simulink model "tapped_delay_line2"  (R2019a)
settings: Solver=FixedStepAuto  StartTime=0.0  StopTime=endtime  FixedStep=0.001  RelTol=1e-3
undefined symbols (not defined in the file or in its folder): Gpd, K
settings Model: Creator=chris  LastModifiedBy=chris

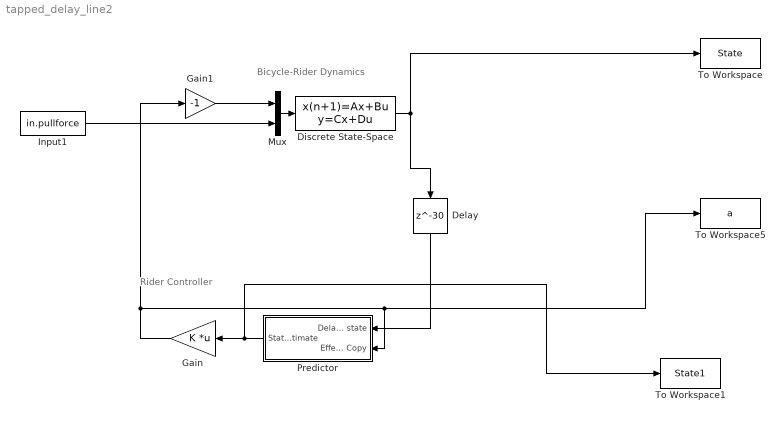
== system tapped_delay_line2 ==
  note: Rider Controller
  note: Bicycle-Rider Dynamics
  Delay : Delay  DelayLength=30  InitialCondition=0
  Discrete State-Space : DiscreteStateSpace  A=Gpd.A  B=Gpd.B  C=Gpd.C  D=Gpd.D  SampleTime=-1
  Gain : Gain  Gain=K  Multiplication=Matrix(K*u) (u vector)
  Gain1 : Gain  Gain=-1
  Input1 : FromWorkspace  VariableName=in.pullforce  SampleTime=0
  Mux : Mux  Inputs=2
  "Predictor " : Subsystem
  To Workspace : ToWorkspace  VariableName=State  SampleTime=-1
  To Workspace1 : ToWorkspace  VariableName=State1  SampleTime=-1
  To Workspace5 : ToWorkspace  VariableName=a  SampleTime=-1
  wires:
  Discrete State-Space/1 -> Delay/1, To Workspace/1
  Mux/1 -> Discrete State-Space/1
  Gain1/1 -> Mux/1
  Input1/1 -> Mux/2
  Gain/1 -> To Workspace5/1, "Predictor "/2("Efference Copy "), Gain1/1
  "Predictor "/1("State Estimate ") -> To Workspace1/1, Gain/1
  Delay/1 -> "Predictor "/1("Delayed state ")

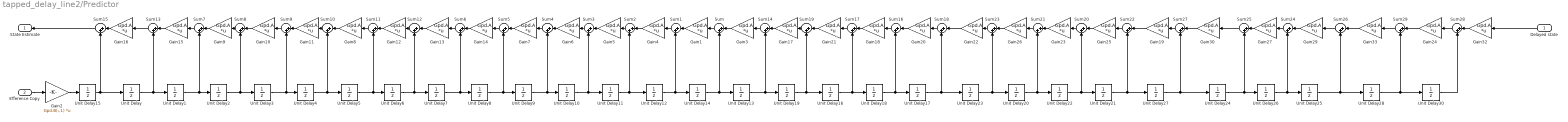
== system tapped_delay_line2/Predictor  ==
  "Delayed state " : Inport
  "Efference Copy " : Inport  Port=2
  Gain{1,3..27,29..30,32..33} (30 alike) : Gain  Gain=Gpd.A  Multiplication=Matrix(K*u) (u vector)
  Gain2 : Gain  Gain=Gpd.B(:,1)  Multiplication=Matrix(K*u) (u vector)
  Sum{,1..29} (30 alike) : Sum  Inputs=|++
  Unit Delay{,1..28,30} (30 alike) : UnitDelay  SampleTime=-1  HasFrameUpgradeWarning=on
  "State Estimate " : Outport
  wires:
  "Efference Copy "/1 -> Gain2/1
  Unit Delay/1 -> Sum13/2, Unit Delay1/1
  Unit Delay1/1 -> Sum7/2, Unit Delay2/1
  Unit Delay2/1 -> Sum8/2, Unit Delay3/1
  Unit Delay3/1 -> Sum9/2, Unit Delay4/1
  Unit Delay4/1 -> Sum10/2, Unit Delay5/1
  Unit Delay5/1 -> Sum11/2, Unit Delay6/1
  Unit Delay6/1 -> Sum12/2, Unit Delay7/1
  Unit Delay7/1 -> Sum6/2, Unit Delay8/1
  Unit Delay8/1 -> Unit Delay9/1, Sum5/2
  Unit Delay9/1 -> Sum4/2, Unit Delay10/1
  Unit Delay10/1 -> Sum3/2, Unit Delay11/1
  Unit Delay11/1 -> Unit Delay12/1, Sum2/2
  Unit Delay14/1 -> Unit Delay13/1, Sum/2
  Unit Delay12/1 -> Sum1/2, Unit Delay14/1
  Gain1/1 -> Sum1/1
  Sum/1 -> Gain1/1
  Gain3/1 -> Sum/1
  Sum1/1 -> Gain4/1
  Sum2/1 -> Gain5/1
  Gain4/1 -> Sum2/1
  Sum3/1 -> Gain6/1
  Gain5/1 -> Sum3/1
  Sum4/1 -> Gain7/1
  Gain6/1 -> Sum4/1
  Sum5/1 -> Gain14/1
  Gain7/1 -> Sum5/1
  Sum6/1 -> Gain13/1
  Gain14/1 -> Sum6/1
  Sum7/1 -> Gain15/1
  Gain9/1 -> Sum7/1
  Sum8/1 -> Gain9/1
  Gain10/1 -> Sum8/1
  Sum9/1 -> Gain10/1
  Gain11/1 -> Sum9/1
  Sum10/1 -> Gain11/1
  Gain8/1 -> Sum10/1
  Sum11/1 -> Gain8/1
  Gain12/1 -> Sum11/1
  Sum12/1 -> Gain12/1
  Gain13/1 -> Sum12/1
  Sum13/1 -> Gain16/1
  Gain15/1 -> Sum13/1
  Unit Delay13/1 -> Sum14/2, Unit Delay19/1
  Sum14/1 -> Gain3/1
  Gain17/1 -> Sum14/1
  Unit Delay15/1 -> Unit Delay/1, Sum15/2
  Gain2/1 -> Unit Delay15/1
  Gain16/1 -> Sum15/1
  Sum15/1 -> "State Estimate "/1
  Unit Delay18/1 -> Unit Delay17/1, Sum16/2
  Gain22/1 -> Sum18/1
  Unit Delay16/1 -> Sum17/2, Unit Delay18/1
  Gain18/1 -> Sum17/1
  Sum17/1 -> Gain21/1
  Sum16/1 -> Gain18/1
  Gain20/1 -> Sum16/1
  Sum18/1 -> Gain20/1
  Unit Delay19/1 -> Unit Delay16/1, Sum19/2
  Sum19/1 -> Gain17/1
  Gain21/1 -> Sum19/1
  Sum20/1 -> Gain23/1
  Sum21/1 -> Gain26/1
  Gain23/1 -> Sum21/1
  Gain25/1 -> Sum20/1
  Unit Delay22/1 -> Unit Delay21/1, Sum20/2
  Unit Delay20/1 -> Sum21/2, Unit Delay22/1
  Gain26/1 -> Sum23/1
  Sum22/1 -> Gain25/1
  Unit Delay23/1 -> Unit Delay20/1, Sum23/2
  Sum23/1 -> Gain22/1
  Unit Delay17/1 -> Unit Delay23/1, Sum18/2
  Gain29/1 -> Sum24/1
  Sum24/1 -> Gain27/1
  Gain33/1 -> Sum26/1
  Unit Delay27/1 -> Unit Delay24/1, Sum27/2
  Unit Delay24/1 -> Sum25/2, Unit Delay26/1
  Sum25/1 -> Gain30/1
  Unit Delay26/1 -> Unit Delay25/1, Sum24/2
  Gain30/1 -> Sum27/1
  Sum26/1 -> Gain29/1
  Sum27/1 -> Gain19/1
  Gain27/1 -> Sum25/1
  Unit Delay21/1 -> Sum22/2, Unit Delay27/1
  Gain19/1 -> Sum22/1
  Unit Delay30/1 -> Sum28/2
  Sum29/1 -> Gain33/1
  Gain24/1 -> Sum29/1
  Unit Delay28/1 -> Unit Delay30/1, Sum29/2
  Unit Delay25/1 -> Unit Delay28/1, Sum26/2
  Gain32/1 -> Sum28/1
  Sum28/1 -> Gain24/1
  "Delayed state "/1 -> Gain32/1
